simulink library "INT_BattU_VD"  (R2016b)
settings: Solver=VariableStepAuto  StartTime=0.0  StopTime=10.0  RelTol=1e-3
settings Model: Creator=xuxingpei  LastModifiedBy=xuxingpei

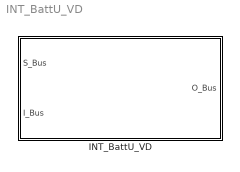
== system INT_BattU_VD ==
  INT_BattU_VD : Subsystem

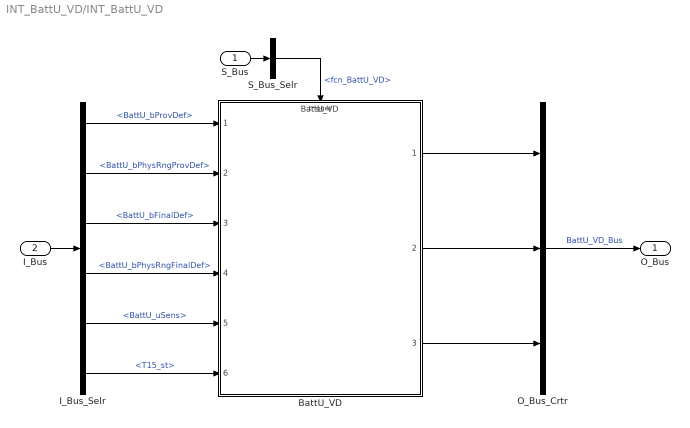
== system INT_BattU_VD/INT_BattU_VD ==
  S_Bus : Inport
  I_Bus : Inport  Port=2
  BattU_VD : ModelReference  ModelNameDialog=BattU_VD  SimulationMode=Normal  ModelReferenceVersion=1.13  TriggerPortName=function  TriggerPortTriggerType=function-call  TriggerPortStatesWhenEnabling=held
  I_Bus_Selr : BusSelector  OutputSignals=BattU_bProvDef,BattU_bPhysRngProvDef,BattU_bFinalDef,BattU_bPhysRngFinalDef,BattU_uSens,T15_st
  O_Bus_Crtr : BusCreator  Inputs=3
  S_Bus_Selr : BusSelector  OutputSignals=fcn_BattU_VD
  O_Bus : Outport
  wires:
  S_Bus_Selr/1 -> BattU_VD/Trigger  "<fcn_BattU_VD>"
  S_Bus/1 -> S_Bus_Selr/1
  I_Bus/1 -> I_Bus_Selr/1
  I_Bus_Selr/1 -> BattU_VD/1  "<BattU_bProvDef>"
  I_Bus_Selr/2 -> BattU_VD/2  "<BattU_bPhysRngProvDef>"
  I_Bus_Selr/3 -> BattU_VD/3  "<BattU_bFinalDef>"
  I_Bus_Selr/4 -> BattU_VD/4  "<BattU_bPhysRngFinalDef>"
  I_Bus_Selr/5 -> BattU_VD/5  "<BattU_uSens>"
  I_Bus_Selr/6 -> BattU_VD/6  "<T15_st>"
  O_Bus_Crtr/1 -> O_Bus/1  "BattU_VD_Bus"
  BattU_VD/1 -> O_Bus_Crtr/1
  BattU_VD/2 -> O_Bus_Crtr/2
  BattU_VD/3 -> O_Bus_Crtr/3
